simulink model "simu_ass1"  (R2025b)
settings: Solver=FixedStepAuto  StartTime=0.0  StopTime=time_10hz(end)  FixedStep=0.1  RelTol=1e-3
values from neighbouring files (symbols this model uses):
  dtheta_int = interp1(pos.time_vect, dtheta, time_10hz)    [ass1_def.m]    (also in assignment1_def.m)
  time_10hz = pos.time_vect(1:5:end)    [ass1_def.m]    (also in assignment1_def.m)
  v_int = interp1(pos.time_vect, v_tot, time_10hz)    [ass1_def.m]    (also in assignment1_def.m)
undefined symbols (not defined in the file or in its folder): Twist
libraries: robotlib x1, ros2lib x1
settings Model: Creator=lucia  LastModifiedBy=lucia

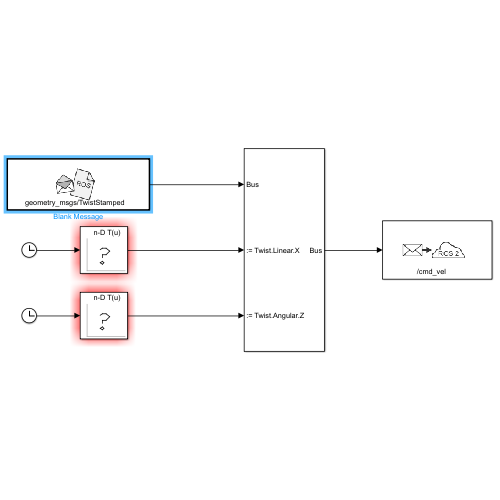
[thumbnail: Simulink's stored preview of the top-level diagram]
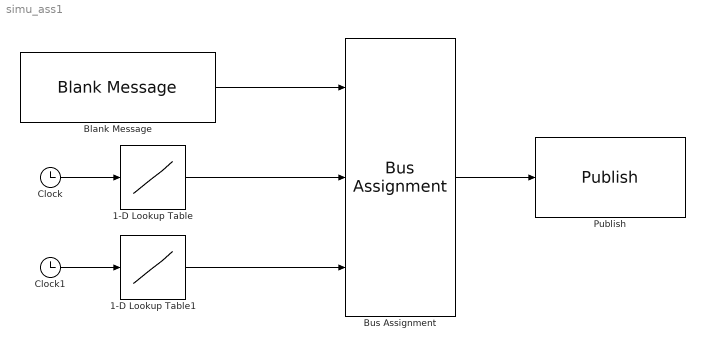
== system simu_ass1 ==
  1-D Lookup Table : Lookup_n-D  NumberOfTableDimensions=1  BreakpointsForDimension1=time_10hz  Table=v_int  InternalRulePriority=Speed  RndMeth=Simplest
  1-D Lookup Table1 : Lookup_n-D  NumberOfTableDimensions=1  BreakpointsForDimension1=time_10hz  Table=dtheta_int  InternalRulePriority=Speed  RndMeth=Simplest
  Blank Message : robotlib/Blank Message  messageClass=Message  entityType=geometry_msgs/TwistStamped  messageType=geometry_msgs/TwistStamped  SampleTime=0.1  legacyBusStruct=off
  Bus Assignment : BusAssignment  AssignedSignals=Twist.Linear.X,Twist.Angular.Z
  Clock : Clock
  Clock1 : Clock
  Publish : ros2lib/Publish  topicSource=Select from ROS network  topic=/cmd_vel  messageType=geometry_msgs/TwistStamped  QOSHistory=Keep last  QOSDepth=10  QOSReliability=Reliable  QOSDurability=Volatile  QOSDeadline=Inf  QOSLifespan=Inf  QOSLiveliness=Automatic  QOSLeaseDuration=Inf  QOSAvoidROSNamespaceConventions=off
  wires:
  Clock/1 -> 1-D Lookup Table/1
  Clock1/1 -> 1-D Lookup Table1/1
  Blank Message/1 -> Bus Assignment/1
  Bus Assignment/1 -> Publish/1
  1-D Lookup Table/1 -> Bus Assignment/2
  1-D Lookup Table1/1 -> Bus Assignment/3
